simulink subsystem "Thruster_Magnitude"  (R2022b)
settings: Solver=VariableStepAuto  StartTime=0.0  StopTime=10.0  RelTol=1e-3
settings Model: Creator=hayden  LastModifiedBy=hollis
settings ModelReferenceCC: EnableRefExpFcnMdlSchedulingChecks=on

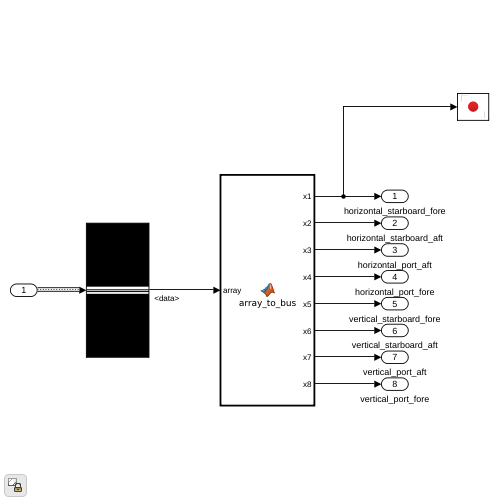
[thumbnail: Simulink's stored preview of the top-level diagram]
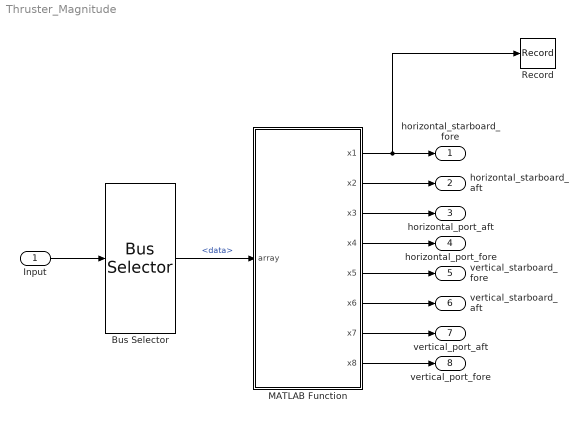
== system Thruster_Magnitude ==
  Input : Inport
  Bus Selector : BusSelector  OutputSignals=data
  MATLAB Function : MATLAB Function  TreatAsAtomicUnit=on
  Record : Record  FileSettingsInternal="{\"entries\":[{\"content\":{\"excelSettings\":{\"content\":{},\"type\":\"Streamout.ExcelSettings\"}},\"type\":\"Streamout.FileSettingStorage\",\"uuid\":\"281036e3-18dc-40ca-bcce-f7e61bc471e7\"}],\"packageUris\":[\"http://schema.mathworks.com/mf0/streamout_blocks/R2020a\"],\"version\":\"1.0\"}"  SignalsInternal="{\"entries\":[{\"content\":{\"signals\":[]},\"type\":\"RecordBlkView.InputSignals\",\"uuid\":\"bdeefeab-0fde-44c6-9a10-550f46accd09\"}],\"packageUris\":[\"http://schema.mathworks.com/mf0/streamout_blocks/R2020a\"],\"version\":\"1.0\"}"  VisualizationBindings="{\"sparklinesplugin\":{\"info\":[{\"bindingParametersList\":[],\"subplotID\":1}]}}"
  horizontal_starboard_fore : Outport
  horizontal_starboard_aft : Outport  Port=2
  horizontal_port_aft : Outport  Port=3
  horizontal_port_fore : Outport  Port=4
  vertical_starboard_fore : Outport  Port=5
  vertical_starboard_aft : Outport  Port=6
  vertical_port_aft : Outport  Port=7
  vertical_port_fore : Outport  Port=8
  wires:
  Bus Selector/1 -> MATLAB Function/1(array)  "<data>"
  MATLAB Function/1(x1) -> horizontal_starboard_fore/1, Record/1
  MATLAB Function/2(x2) -> horizontal_starboard_aft/1
  MATLAB Function/3(x3) -> horizontal_port_aft/1
  MATLAB Function/4(x4) -> horizontal_port_fore/1
  MATLAB Function/5(x5) -> vertical_starboard_fore/1
  MATLAB Function/6(x6) -> vertical_starboard_aft/1
  MATLAB Function/7(x7) -> vertical_port_aft/1
  MATLAB Function/8(x8) -> vertical_port_fore/1
  Input/1 -> Bus Selector/1

== matlab function Thruster_Magnitude/MATLAB Function ==
  data: array input; x1 output; x2 output; x3 output; x4 output; x5 output; x6 output; x7 output; x8 output
function [x1,x2,x3,x4,x5,x6,x7,x8] = array_to_bus(array)

    x1 = array(1);
    x2 = array(2);
    x3 = array(3);
    x4 = array(4);
    x5 = array(5);
    x6 = array(6);
    x7 = array(7);
    x8 = array(8);
end
